simulink model "Sens_UltraStick120"  (R2016b)
settings: Solver=VariableStepAuto  StartTime=0.0  StopTime=10.0  RelTol=1e-3
undefined symbols (not defined in the file): AC
libraries: SensLib x4, OpenFlightUtilLib x1
settings Model: Creator=UAVLAB  LastModifiedBy=rega0051

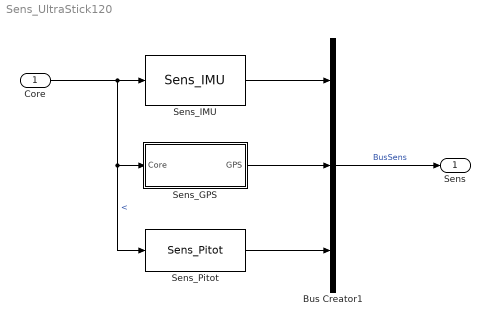
== system Sens_UltraStick120 ==
  Core : Inport  OutDataTypeStr=Bus: BusCore
  Bus Creator1 : BusCreator  Inputs=3  OutDataTypeStr=Bus: BusSens
      settings: AttributesFormatString=%<OutDataTypeStr>  InheritFromInputs=off
  Sens_GPS : Subsystem  AncestorBlock=SensLib/Sens_GPS  TreatAsAtomicUnit=on  VariantControl=Variant1  mask{sens=AC.Sens.GPS}
      mask prompts: sens "GPS Parameter Structure:"
  Sens_IMU : SensLib/Sens_IMU  VariantControl=VarImu_LocTransErr  sens=AC.Sens.IMU
  Sens_Pitot : SensLib/Sens_Pitot  VariantControl=VarAirData_LocTransErr  sens=AC.Sens.AirData
  Sens : Outport  OutDataTypeStr=Bus: BusSens
  wires:
  Core/1 -> Sens_GPS/1(Core), Sens_Pitot/1, Sens_IMU/1  "<"
  Bus Creator1/1 -> Sens/1  "BusSens"
  Sens_GPS/1(GPS) -> Bus Creator1/2
  Sens_Pitot/1 -> Bus Creator1/3
  Sens_IMU/1 -> Bus Creator1/1

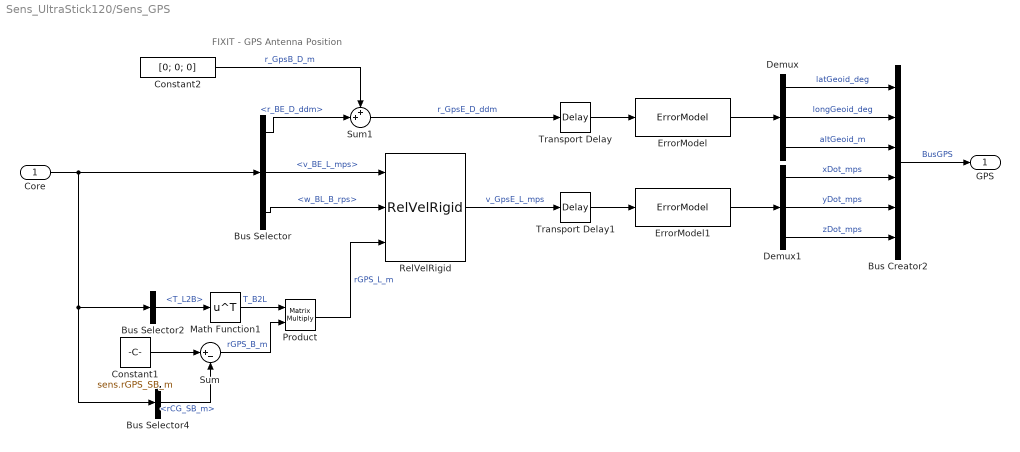
== system Sens_UltraStick120/Sens_GPS ==
  note: FIXIT - GPS Antenna Position
  Core : Inport
  Bus Creator2 : BusCreator  Inputs=6  OutDataTypeStr=Bus: BusGPS
      settings: InheritFromInputs=off
  Bus Selector : BusSelector  OutputSignals=BusEom.r_BE_D_ddm,BusEom.v_BE_L_mps,BusEom.w_BL_B_rps
  Bus Selector2 : BusSelector  OutputSignals=BusEom.T_L2B
  Bus Selector4 : BusSelector  OutputSignals=BusEom.rCG_SB_m
  Constant1 : Constant  Value=sens.rGPS_SB_m
      settings: AttributesFormatString=%<Value>
  Constant2 : Constant  Value=[0; 0; 0]
      settings: AttributesFormatString=%<Value>
  Demux : Demux  Outputs=3
  Demux1 : Demux  Outputs=3
  ErrorModel : SensLib/ErrorModel  enable=sens.errEnable  scf=sens.posScf  bias=sens.posBias  sigma=sens.posSigma  seed=sens.posSeed  timestep=sens.timeSample_s
  ErrorModel1 : SensLib/ErrorModel  enable=sens.errEnable  scf=sens.velScf  bias=sens.velBias  sigma=sens.velSigma  seed=sens.velSeed  timestep=sens.timeSample_s
  Math Function1 : Math  Operator=transpose  SaturateOnIntegerOverflow=on
  Product : Product  Multiplication=Matrix(*)
  RelVelRigid : OpenFlightUtilLib/Kinematics and Dynamics/RelVelRigid
  Sum : Sum  Inputs=|+-
  Sum1 : Sum  Inputs=++|
  Transport Delay : TransportDelay  DelayTime=sens.timeDelay_s  TransDelayFeedthrough=on  PadeOrder=2
      settings: AttributesFormatString=%<DelayTime>
  Transport Delay1 : TransportDelay  DelayTime=sens.timeDelay_s  TransDelayFeedthrough=on  PadeOrder=2
      settings: AttributesFormatString=%<DelayTime>
  GPS : Outport
  wires:
  Core/1 -> Bus Selector4/1, Bus Selector2/1, Bus Selector/1
  Demux/2 -> Bus Creator2/2  "longGeoid_deg"
  Demux/1 -> Bus Creator2/1  "latGeoid_deg"
  Demux/3 -> Bus Creator2/3  "altGeoid_m"
  Bus Selector/3 -> RelVelRigid/2  "<w_BL_B_rps>"
  Bus Creator2/1 -> GPS/1  "BusGPS"
  Demux1/1 -> Bus Creator2/4  "xDot_mps"
  Demux1/2 -> Bus Creator2/5  "yDot_mps"
  Demux1/3 -> Bus Creator2/6  "zDot_mps"
  ErrorModel/1 -> Demux/1
  ErrorModel1/1 -> Demux1/1
  Constant1/1 -> Sum/1
  Sum/1 -> Product/2  "rGPS_B_m"
  Bus Selector/1 -> Sum1/2  "<r_BE_D_ddm>"
  Sum1/1 -> Transport Delay/1  "r_GpsE_D_ddm"
  RelVelRigid/1 -> Transport Delay1/1  "v_GpsE_L_mps"
  Transport Delay/1 -> ErrorModel/1
  Transport Delay1/1 -> ErrorModel1/1
  Bus Selector4/1 -> Sum/2  "<rCG_SB_m>"
  Bus Selector/2 -> RelVelRigid/1  "<v_BE_L_mps>"
  Bus Selector2/1 -> Math Function1/1  "<T_L2B>"
  Math Function1/1 -> Product/1  "T_B2L"
  Product/1 -> RelVelRigid/3  "rGPS_L_m"
  Constant2/1 -> Sum1/1  "r_GpsB_D_m"
